simulink model "backstepping"  (R2025a)
settings: Solver=ode4  StartTime=0.0  StopTime=t_total(end)  RelTol=1e-3
StopFcn:
  | autoplot;
values from neighbouring files (symbols this model uses):
  Ib = diag([params.Ix, params.Iy, params.Iz])    [setup_mission.m]
  lin_vel_0 = [0; 0; 0]    [setup_mission.m]
  mass = params.m    [setup_mission.m]
  pos_0 = p_ref(:,1) + offset_init    [setup_mission.m]
  w_bb_0 = [0; 0; 0]    [setup_mission.m]
libraries: robotcorelib x2, uavutilslib x1
settings Model: Creator=marco  LastModifiedBy=marco

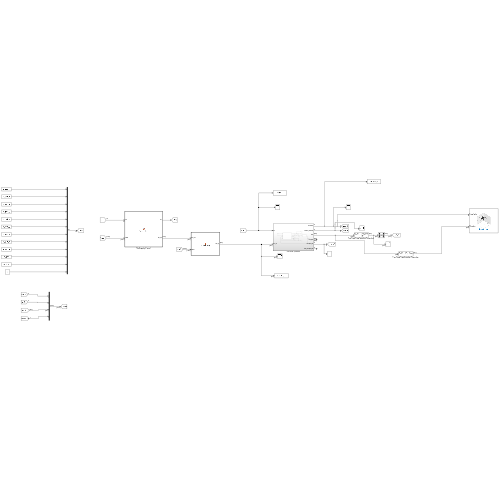
[thumbnail: Simulink's stored preview of the top-level diagram]
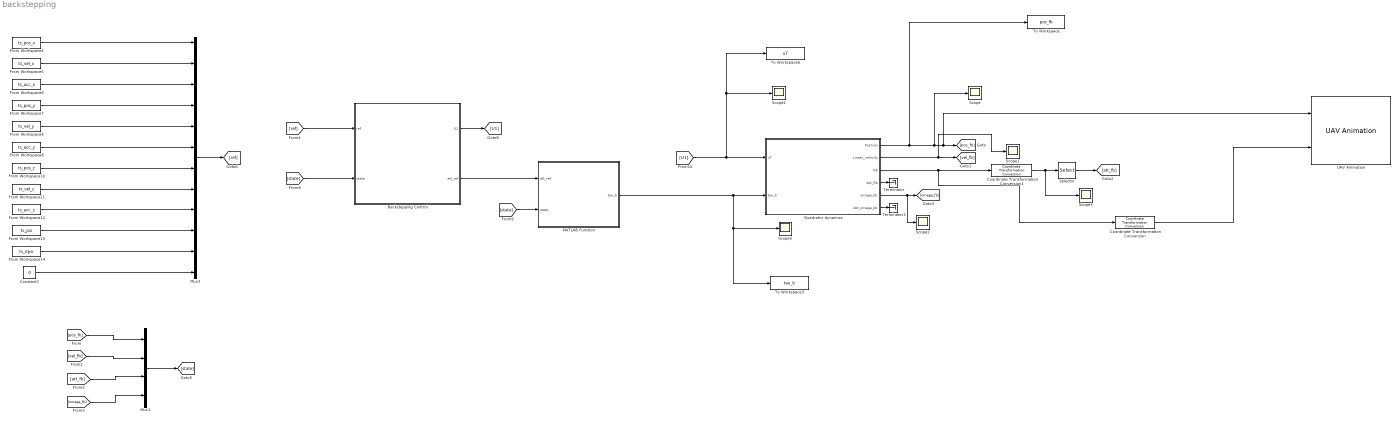
== system backstepping ==
  Backstepping Control : MATLAB Function  TreatAsAtomicUnit=on
  Constant7 : Constant  Value=0
  Coordinate Transformation Conversion : robotcorelib/Coordinate Transformation Conversion  InputRepresentation=Rotation Matrix  InputEulerSequence=ZYX  ShowTrVecInputPort=on  OutputRepresentation=Quaternion  OutputEulerSequence=ZYX  ShowTrVecOutputPort=on  SimulateUsing=Interpreted execution
  Coordinate Transformation Conversion1 : robotcorelib/Coordinate Transformation Conversion  InputRepresentation=Rotation Matrix  InputEulerSequence=ZYX  ShowTrVecInputPort=on  OutputRepresentation=Euler Angles  OutputEulerSequence=ZYX  ShowTrVecOutputPort=on  SimulateUsing=Interpreted execution
  From Workspace10 : FromWorkspace  VariableName=ts_pos_z
  From Workspace11 : FromWorkspace  VariableName=ts_vel_z
  From Workspace12 : FromWorkspace  VariableName=ts_acc_z
  From Workspace13 : FromWorkspace  VariableName=ts_psi
  From Workspace14 : FromWorkspace  VariableName=ts_dpsi
  From Workspace4 : FromWorkspace  VariableName=ts_pos_x
  From Workspace5 : FromWorkspace  VariableName=ts_vel_x
  From Workspace6 : FromWorkspace  VariableName=ts_acc_x
  From Workspace7 : FromWorkspace  VariableName=ts_pos_y
  From Workspace8 : FromWorkspace  VariableName=ts_acc_y
  From Workspace9 : FromWorkspace  VariableName=ts_vel_y
  MATLAB Function : MATLAB Function  TreatAsAtomicUnit=on
  Mux1 : Mux
  Mux3 : Mux  Inputs=12
  Quadrotor dynamics : Subsystem
  Scope{,1..5} (6 alike) : Scope
      Scope settings: ActiveDisplayYMinimum=-4.6326382236688541  ActiveDisplayYMaximum=1.6258456698835591
      Scope1 settings: ActiveDisplayYMinimum=-2.7724427496717432  ActiveDisplayYMaximum=2.7786427222497823
      Scope2 settings: ActiveDisplayYMinimum=-0.39873826993187278  ActiveDisplayYMaximum=0.30941670916189168  DataLoggingVariableName=ScopeData2
      Scope3 settings: ActiveDisplayYMinimum=-0.19912218673134091  ActiveDisplayYMaximum=0.1796006205396169  DataLoggingVariableName=ScopeData3
      Scope4 settings: ActiveDisplayYMinimum=11.687086404838853  ActiveDisplayYMaximum=11.856708503122613  DataLoggingVariableName=ScopeData4
      Scope5 settings: ActiveDisplayYMinimum=-0.020164289135421433  ActiveDisplayYMaximum=0.020163735646024  DataLoggingVariableName=ScopeData5
  Selector : Selector  InputPortWidth=3  IndexOptions=Index vector (dialog)  Indices=[3, 2, 1]  OutputSizes=1
  Terminator : Terminator
  Terminator3 : Terminator
  To Workspace : ToWorkspace  VariableName=pos_fb  SaveFormat=Timeseries  SampleTime=-1
  To Workspace3 : ToWorkspace  VariableName=tau_b  SaveFormat=Timeseries  SampleTime=-1
  To Workspace6 : ToWorkspace  VariableName=uT  SaveFormat=Timeseries  SampleTime=-1
  UAV Animation : uavutilslib/UAV Animation  NumUAV=1  DynamicUAVConfig=off  UAVType=Multirotor  UAVSize=1  UAVColor=[1 0 0]  UAVTrajectoryAlpha=1  InertialZDirection=Down  RotationFormat=Quaternion  DrawMarkers=off  SampleTime=0.01
  wires:
  Quadrotor dynamics/4(dot_Rb) -> Terminator/1
  Quadrotor dynamics/2(Linear_velocity) -> Scope1/1, [vel_fb]
  Quadrotor dynamics/6(dot_omega_bb) -> Terminator3/1
  Quadrotor dynamics/1(Position) -> To Workspace/1, Scope/1, UAV Animation/1, [pos_fb]
  Quadrotor dynamics/5(omega_bb) -> [omega_fb], Scope2/1
  Quadrotor dynamics/3(Rb) -> Coordinate Transformation Conversion/1, Coordinate Transformation Conversion1/1
  Coordinate Transformation Conversion1/1 -> Selector/1, Scope3/1
  [omega_fb] -> Mux1/4
  [att_fb] -> Mux1/3
  [vel_fb] -> Mux1/2
  [pos_fb] -> Mux1/1
  Selector/1 -> [att_fb]
  MATLAB Function/1(tau_b) -> To Workspace3/1, Scope5/1, Quadrotor dynamics/2(tau_b)
  Mux3/1 -> [ref]
  From Workspace7/1 -> Mux3/4
  Constant7/1 -> Mux3/12
  From Workspace8/1 -> Mux3/6
  From Workspace14/1 -> Mux3/11
  From Workspace13/1 -> Mux3/10
  From Workspace12/1 -> Mux3/9
  From Workspace11/1 -> Mux3/8
  From Workspace10/1 -> Mux3/7
  From Workspace9/1 -> Mux3/5
  From Workspace4/1 -> Mux3/1
  From Workspace6/1 -> Mux3/3
  From Workspace5/1 -> Mux3/2
  [ref] -> Backstepping Control/1(ref)
  Mux1/1 -> [state]
  [state] -> Backstepping Control/2(state)
  Backstepping Control/1(U1) -> [U1]
  Coordinate Transformation Conversion/1 -> UAV Animation/2
  Backstepping Control/2(att_ref) -> MATLAB Function/1(att_ref)
  [state] -> MATLAB Function/2(state)
  [U1] -> Scope4/1, To Workspace6/1, Quadrotor dynamics/1(uT)

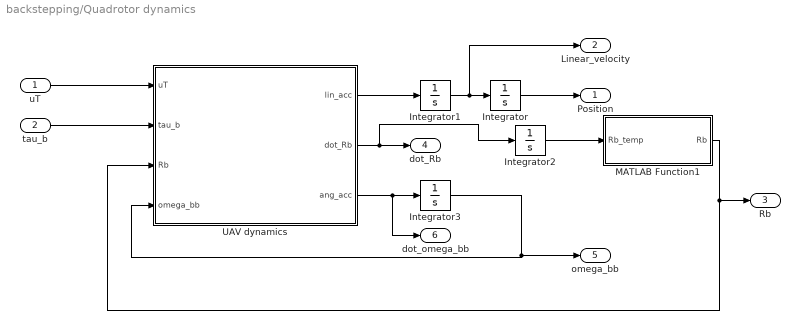
== system backstepping/Quadrotor dynamics ==
  uT : Inport
  tau_b : Inport  Port=2
  Integrator : Integrator  InitialCondition=pos_0
  Integrator1 : Integrator  InitialCondition=lin_vel_0
  Integrator2 : Integrator  InitialCondition=[1 0 0; 0 1 0;0 0 1]
  Integrator3 : Integrator  InitialCondition=w_bb_0
  MATLAB Function1 : MATLAB Function  TreatAsAtomicUnit=on
  UAV dynamics : MATLAB Function  TreatAsAtomicUnit=on
  Position : Outport
  Linear_velocity : Outport  Port=2
  Rb : Outport  Port=3
  dot_Rb : Outport  Port=4
  omega_bb : Outport  Port=5
  dot_omega_bb : Outport  Port=6
  wires:
  tau_b/1 -> UAV dynamics/2(tau_b)
  Integrator/1 -> Position/1
  UAV dynamics/3(ang_acc) -> dot_omega_bb/1, Integrator3/1
  UAV dynamics/1(lin_acc) -> Integrator1/1
  uT/1 -> UAV dynamics/1(uT)
  Integrator1/1 -> Linear_velocity/1, Integrator/1
  Integrator3/1 -> UAV dynamics/4(omega_bb), omega_bb/1
  UAV dynamics/2(dot_Rb) -> Integrator2/1, dot_Rb/1
  MATLAB Function1/1(Rb) -> Rb/1, UAV dynamics/3(Rb)
  Integrator2/1 -> MATLAB Function1/1(Rb_temp)

== matlab function backstepping/Quadrotor dynamics/UAV dynamics ==
  data: uT input size=1; tau_b input size=3; lin_acc output size=3; Rb input size=[3,3]; omega_bb input size=3; dot_Rb output size=[3,3]; ang_acc output size=3; mass parameter size=1; Ib parameter size=[3,3]
function [lin_acc, dot_Rb, ang_acc] = fcn(uT,tau_b,Rb,omega_bb,mass, Ib)

lin_acc = 9.81*[0 0 1]'-(uT/mass)*Rb*[0 0 1]';
dot_Rb = Rb*skew(omega_bb);
ang_acc = inv(Ib)*(-skew(omega_bb)*Ib*omega_bb + tau_b);

end

function S = skew(v)
if(numel(v)~= 1)
S= [0 -v(3) v(2); 
    v(3) 0 -v(1);
    -v(2) v(1) 0];
else
S= zeros(3);
end
end

== matlab function backstepping/Backstepping Control ==
  data: ref input; U1 output; state input; params parameter; att_ref output
function [U1, att_ref] = bs_outer_loop(ref, state, params)
% --- BACKSTEPPING OUTER LOOP (POSITION) ---
% ref structure: [x,vx,ax, y,vy,ay, z,vz,az, psi,dpsi,ddpsi]

% --- STATE EXTRACTION ---
x = state(1); y = state(2); z = state(3);
vx = state(4); vy = state(5); vz = state(6);
psi = state(9); % Necessary to rotate the desired force

m = params.m; 
g = 9.81; 

% --- REFERENCE EXTRACTION ---
x_d  = ref(1); vx_d = ref(2); ax_d = ref(3);
y_d  = ref(4); vy_d = ref(5); ay_d = ref(6);
z_d  = ref(7); vz_d = ref(8); az_d = ref(9);
psi_d   = ref(10); dpsi_d  = ref(11);

pos_d = [x_d; y_d; z_d];
vel_d = [vx_d; vy_d; vz_d];
acc_d = [ax_d; ay_d; az_d];

pos_act = [x; y; z];
vel_act = [vx; vy; vz];

% --- GAIN TUNING ---
Kp = [6.0; 6.0; 20.0];    
Kd = [4.5; 4.5; 12.0];    

e_pos = pos_d - pos_act;
e_vel = vel_d - vel_act;

% Desired acceleration
acc_des = acc_d + Kp .* e_pos + Kd .* e_vel;

% Total Inertial Force
g_vec = [0; 0; 9.81];
F_des_inertial = m * (acc_des - g_vec); 

% --- (Total Thrust) ---
U1 = norm(F_des_inertial);
U1 = max(1.0, min(25, U1)); % Saturation

% --- DESIRED ANGLES EXTRACTION ---
R_psi = [cos(psi) -sin(psi) 0;
         sin(psi)  cos(psi) 0;
         0         0        1];

F_body_intermediate = R_psi' * F_des_inertial; 
Fx_cmd = F_body_intermediate(1);
Fy_cmd = F_body_intermediate(2);

% Angles Calculation
theta_d = asin(-Fx_cmd / U1);
phi_d = asin(Fy_cmd / (U1 * cos(theta_d)));

% Angles Saturation
lim_ang = 0.6; 
theta_d = max(-lim_ang, min(lim_ang, theta_d));
phi_d   = max(-lim_ang, min(lim_ang, phi_d));

% Complex numbers check for safety
if ~isreal(theta_d), theta_d = 0; end
if ~isreal(phi_d), phi_d = 0; end

% --- OUTPUT ---
att_ref = [phi_d; theta_d; psi_d; dpsi_d];
end

== matlab function backstepping/MATLAB Function ==
  data: att_ref input; tau_b output; state input; params parameter
function tau_b  = bs_inner_loop(att_ref, state, params)
% --- BACKSTEPPING INNER LOOP (ATTITUDE) ---

% --- DATA EXTRACTION ---
phi_d   = att_ref(1);
theta_d = att_ref(2);
psi_d   = att_ref(3);
dpsi_d  = att_ref(4);

% Current drone state
phi = state(7); theta = state(8); psi = state(9);
p = state(10); q = state(11); r = state(12);

Ix = params.Ix; Iy = params.Iy; Iz = params.Iz;

% --- GAIN TUNING ---
K_att  = [70; 70; 40];    
K_rate = [18; 18; 14];    

% --- ERROR CALCULATION ---
e_phi   = phi_d - phi;
e_theta = theta_d - theta;
e_psi   = psi_d - psi;

de_phi   = 0 - p;       
de_theta = 0 - q;
de_psi   = dpsi_d - r;  

% --- CONTROL TORQUES CALCULATION ---
tau_phi   = Ix * (K_att(1) * e_phi   + K_rate(1) * de_phi);
tau_theta = Iy * (K_att(2) * e_theta + K_rate(2) * de_theta);
tau_psi   = Iz * (K_att(3) * e_psi   + K_rate(3) * de_psi);

% --- OUTPUT ---
% Torques vector (U2, U3, U4)
tau_b = [tau_phi; tau_theta; tau_psi];

end

== matlab function backstepping/Quadrotor dynamics/MATLAB Function1 ==
  data: Rb_temp input; Rb output
function Rb = fcn(Rb_temp)
    [U,S,V] = svd(Rb_temp);
    sigma = det(U*V');
    S_ = diag([1 1 sigma]);

    Rb = U*S_*V';
end
